simulink model "LateralControlDesignWashoutSystem"  (R2020b)
settings: Solver=ode15s  StartTime=0.0  StopTime=100  RelTol=1e-3
values from neighbouring files (symbols this model uses):
  actuatorDen = [1,   actuatorTimeConstant]    [LateralControl.m]    (also in LongitudinalControl.m)
  actuatorNum = actuatorGain*actuatorTimeConstant    (= 5)    [LateralControl.m]    (also in LongitudinalControl.m)
  DGain = PGain*Td    (= 0.156)    [LateralControl.m]    (also in LongitudinalControl.m = 0.0211)
  PGain = 1.56    [LateralControl.m]    (also in LongitudinalControl.m = 0.211)
  stepCommand = 0    [LateralControl.m]    (also in LongitudinalControl.m = 1)
undefined symbols (not defined in the file or in its folder): ALatWashOut, BLatWashOut, CLatWashOut, DLatWashOut, FRoll, FWashOut, InitialConditionsWashOut
libraries: slpidlib x2
settings Model: Creator=Antonis Kantounias  LastModifiedBy=Antonis Kantounias

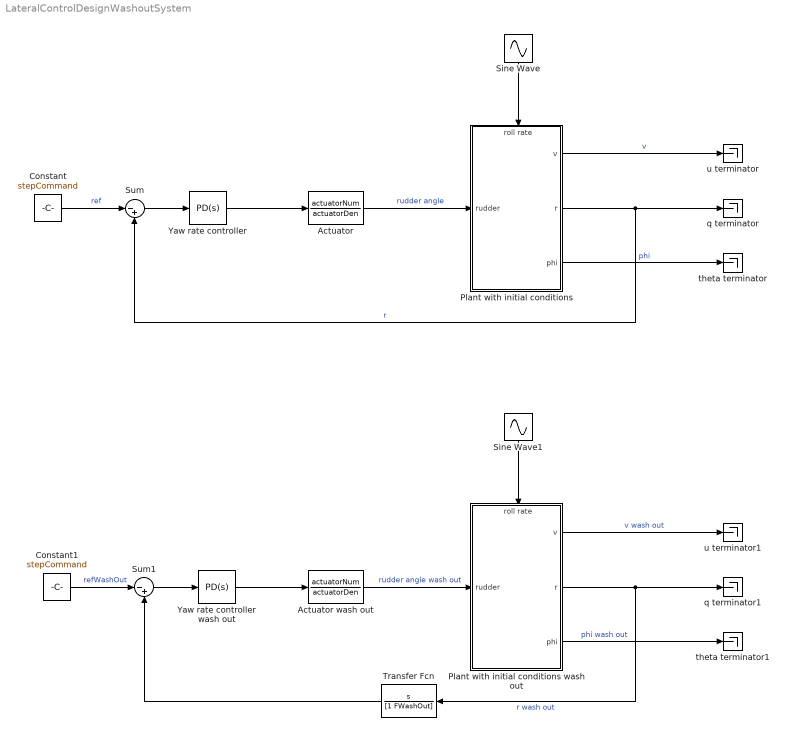
== system LateralControlDesignWashoutSystem ==
  Actuator : TransferFcn  Numerator=actuatorNum  Denominator=actuatorDen
  Actuator wash out : TransferFcn  Numerator=actuatorNum  Denominator=actuatorDen
  Constant : Constant  Value=stepCommand
  Constant1 : Constant  Value=stepCommand
  Plant with initial conditions : Subsystem
      settings: PortSchema="{\"entries\":[{\"content\":{\"sides\":[{\"content\":{\"connectorIds\":[\"In1\"]},\"type\":\"ConnectorPlacement.EquallySpacedRectSide\",\"uuid\":\"9289d697-068e-4568-8078-07f153e8e6b2\"},{\"content\":{\"connectorIds\":[\"Out1\",\"Out2\",\"Out3\"],\"side\":\"RIGHT\"},\"type\":\"ConnectorPlacement.EquallySpacedRectSide\",\"uuid\":\"07e3031a-d198-40ae-947d-4a1b1bfc261d\"},{\"content\":{\"connectorIds\":[\"In2\"],\"side\":\"TOP\"},\"type\":\"ConnectorPlacement.EquallySpacedRectSide\",\"uuid\":\"5510f47b-c9e9-4254-80f0-6c17108d1080\"},{\"content\":{\"connectorIds\":[],\"side\":\"HIDDEN\"},\"type\":\"ConnectorPlacement.EquallySpacedRectSide\",\"uuid\":\"028157a7-30e9-47c8-8173-f7276b1e18d8\"}]},\"type\":\"ConnectorPlacement.EquallySpacedConnector\",\"uuid\":\"3949036d-ff12-4955-8ea8-3a5b06263006\"}],\"packageUris\":[\"http://schema.mathworks.com/mf0/Connector/R2020b\"],\"version\":\"1.0\"}"
  Plant with initial conditions wash out : Subsystem
      settings: PortSchema="{\"entries\":[{\"content\":{\"sides\":[{\"content\":{\"connectorIds\":[\"In1\"]},\"type\":\"ConnectorPlacement.EquallySpacedRectSide\",\"uuid\":\"9289d697-068e-4568-8078-07f153e8e6b2\"},{\"content\":{\"connectorIds\":[\"Out1\",\"Out2\",\"Out3\"],\"side\":\"RIGHT\"},\"type\":\"ConnectorPlacement.EquallySpacedRectSide\",\"uuid\":\"07e3031a-d198-40ae-947d-4a1b1bfc261d\"},{\"content\":{\"connectorIds\":[\"In2\"],\"side\":\"TOP\"},\"type\":\"ConnectorPlacement.EquallySpacedRectSide\",\"uuid\":\"5510f47b-c9e9-4254-80f0-6c17108d1080\"},{\"content\":{\"connectorIds\":[],\"side\":\"HIDDEN\"},\"type\":\"ConnectorPlacement.EquallySpacedRectSide\",\"uuid\":\"028157a7-30e9-47c8-8173-f7276b1e18d8\"}]},\"type\":\"ConnectorPlacement.EquallySpacedConnector\",\"uuid\":\"3949036d-ff12-4955-8ea8-3a5b06263006\"}],\"packageUris\":[\"http://schema.mathworks.com/mf0/Connector/R2020b\"],\"version\":\"1.0\"}"
  Sine Wave : Sin  Frequency=FRoll  SampleTime=0
  Sine Wave1 : Sin  Frequency=FRoll  SampleTime=0
  Sum : Sum  Inputs=|-+
  Sum1 : Sum  Inputs=|-+
  Transfer Fcn : TransferFcn  Numerator=[1,0]  Denominator=[1 FWashOut]
  Yaw rate controller : slpidlib/PID Controller  Controller=PD  Form=Parallel  TimeDomain=Continuous-time  UseExternalTs=off  SampleTime=-1  IntegratorMethod=Forward Euler  FilterMethod=Forward Euler  ControllerParametersSource=internal  P=PGain  I=1  D=DGain  UseFilter=on  N=50  TunerSelectOption=Transfer Function Based (PID Tuner App)  InitialConditionSource=internal  InitialConditionForIntegrator=0  InitialConditionForFilter=0  DifferentiatorICPrevScaledInput=0  ExternalReset=none  TrackingMode=off  Kt=1  LimitOutput=off  SatLimitsSource=internal  UpperSaturationLimit=inf  LowerSaturationLimit=-inf  LinearizeAsGain=on  AntiWindupMode=none  Kb=1  POutMin=[]  POutMax=[]  IOutMin=[]  IOutMax=[]  DOutMin=[]  DOutMax=[]  NOutMin=[]  NOutMax=[]  SumOutMin=[]  SumOutMax=[]  SaturationOutMin=[]  SaturationOutMax=[]  PParamMin=[]  PParamMax=[]  IParamMin=[]  IParamMax=[]  DParamMin=[]  DParamMax=[]  NParamMin=[]  NParamMax=[]  KbParamMin=[]  KbParamMax=[]  KtParamMin=[]  KtParamMax=[]  KbOutMin=[]  KbOutMax=[]  KtOutMin=[]  KtOutMax=[]  IntegratorOutMin=[]  IntegratorOutMax=[]  FilterOutMin=[]  FilterOutMax=[]  SumI1OutMin=[]  SumI1OutMax=[]  SumI2OutMin=[]  SumI2OutMax=[]  SumI3OutMin=[]  SumI3OutMax=[]  SumI4OutMin=[]  SumI4OutMax=[]  SumDOutMin=[]  SumDOutMax=[]  DifferentiatorOutMin=[]  DifferentiatorOutMax=[]  FilterDiffOutCoefMin=[]  FilterDiffOutCoefMax=[]  ReciprocalOutMin=[]  ReciprocalOutMax=[]  SumDenOutMin=[]  SumDenOutMax=[]  SumNumOutMin=[]  SumNumOutMax=[]  DivideOutMin=[]  DivideOutMax=[]  UdiffTsProdOutMin=[]  UdiffTsProdOutMax=[]  NTsProdOutMin=[]  NTsProdOutMax=[]  UintegralTsProdOutMin=[]  UintegralTsProdOutMax=[]  UngainTsProdOutMin=[]  UngainTsProdOutMax=[]  IntegratorContinuousStateAttributes=''  IntegratorStateMustResolveToSignalObject=off  IntegratorRTWStateStorageClass=Auto  FilterContinuousStateAttributes=''  FilterStateMustResolveToSignalObject=off  FilterRTWStateStorageClass=Auto  ParallelPVariant=InternalParameters  IdealPVariant=Disabled  IVariant=Disabled  DVariant=InternalParameters  IntegratorVariant=Disabled  SatVariant=Disabled  AWVariant=Disabled  PCopyVariant=Disabled  TRVariant=Disabled  FdbkBlocksVariant=Forward  IdealPFdbkVariant=Disabled  SatFdbkVariant=Disabled  DerivativeFilterVariant=ContFilter  NVariant=InternalParameters  NCopyVariant=Disabled  FilterICVariant=InternalICsFilter  IntegratorICVariant=Disabled  ExternalResetVariant=Disabled  TRSumVariant=Passthrough  SumFdbkVariant=Disabled  SumVariant=Sum_PD  TsampFilterVariant=InternalTs  TsampNgainVariant=Passthrough  TsampIntegralVariant=Disabled_SignalSpec  ExternalSaturationOutDataTypeStr=Inherit: Same as second input
  "Yaw rate controller wash out " : slpidlib/PID Controller  Controller=PD  Form=Parallel  TimeDomain=Continuous-time  UseExternalTs=off  SampleTime=-1  IntegratorMethod=Forward Euler  FilterMethod=Forward Euler  ControllerParametersSource=internal  P=PGain  I=1  D=DGain  UseFilter=on  N=50  TunerSelectOption=Transfer Function Based (PID Tuner App)  InitialConditionSource=internal  InitialConditionForIntegrator=0  InitialConditionForFilter=0  DifferentiatorICPrevScaledInput=0  ExternalReset=none  TrackingMode=off  Kt=1  LimitOutput=off  SatLimitsSource=internal  UpperSaturationLimit=inf  LowerSaturationLimit=-inf  LinearizeAsGain=on  AntiWindupMode=none  Kb=1  POutMin=[]  POutMax=[]  IOutMin=[]  IOutMax=[]  DOutMin=[]  DOutMax=[]  NOutMin=[]  NOutMax=[]  SumOutMin=[]  SumOutMax=[]  SaturationOutMin=[]  SaturationOutMax=[]  PParamMin=[]  PParamMax=[]  IParamMin=[]  IParamMax=[]  DParamMin=[]  DParamMax=[]  NParamMin=[]  NParamMax=[]  KbParamMin=[]  KbParamMax=[]  KtParamMin=[]  KtParamMax=[]  KbOutMin=[]  KbOutMax=[]  KtOutMin=[]  KtOutMax=[]  IntegratorOutMin=[]  IntegratorOutMax=[]  FilterOutMin=[]  FilterOutMax=[]  SumI1OutMin=[]  SumI1OutMax=[]  SumI2OutMin=[]  SumI2OutMax=[]  SumI3OutMin=[]  SumI3OutMax=[]  SumI4OutMin=[]  SumI4OutMax=[]  SumDOutMin=[]  SumDOutMax=[]  DifferentiatorOutMin=[]  DifferentiatorOutMax=[]  FilterDiffOutCoefMin=[]  FilterDiffOutCoefMax=[]  ReciprocalOutMin=[]  ReciprocalOutMax=[]  SumDenOutMin=[]  SumDenOutMax=[]  SumNumOutMin=[]  SumNumOutMax=[]  DivideOutMin=[]  DivideOutMax=[]  UdiffTsProdOutMin=[]  UdiffTsProdOutMax=[]  NTsProdOutMin=[]  NTsProdOutMax=[]  UintegralTsProdOutMin=[]  UintegralTsProdOutMax=[]  UngainTsProdOutMin=[]  UngainTsProdOutMax=[]  IntegratorContinuousStateAttributes=''  IntegratorStateMustResolveToSignalObject=off  IntegratorRTWStateStorageClass=Auto  FilterContinuousStateAttributes=''  FilterStateMustResolveToSignalObject=off  FilterRTWStateStorageClass=Auto  ParallelPVariant=InternalParameters  IdealPVariant=Disabled  IVariant=Disabled  DVariant=InternalParameters  IntegratorVariant=Disabled  SatVariant=Disabled  AWVariant=Disabled  PCopyVariant=Disabled  TRVariant=Disabled  FdbkBlocksVariant=Forward  IdealPFdbkVariant=Disabled  SatFdbkVariant=Disabled  DerivativeFilterVariant=ContFilter  NVariant=InternalParameters  NCopyVariant=Disabled  FilterICVariant=InternalICsFilter  IntegratorICVariant=Disabled  ExternalResetVariant=Disabled  TRSumVariant=Passthrough  SumFdbkVariant=Disabled  SumVariant=Sum_PD  TsampFilterVariant=InternalTs  TsampNgainVariant=Passthrough  TsampIntegralVariant=Disabled_SignalSpec  ExternalSaturationOutDataTypeStr=Inherit: Same as second input
  q terminator : Terminator
  q terminator1 : Terminator
  theta terminator : Terminator
  theta terminator1 : Terminator
  u terminator : Terminator
  u terminator1 : Terminator
  wires:
  Plant with initial conditions/2(r) -> q terminator/1, Sum/2  "r"
  Plant with initial conditions/1(v) -> u terminator/1  "v"
  Plant with initial conditions/3(phi) -> theta terminator/1  "phi"
  Constant/1 -> Sum/1  "ref"
  Sum/1 -> Yaw rate controller/1
  Yaw rate controller/1 -> Actuator/1
  Actuator/1 -> Plant with initial conditions/1(rudder)  "rudder angle"
  Sine Wave/1 -> Plant with initial conditions/2(roll rate)
  Sine Wave1/1 -> Plant with initial conditions wash out/2(roll rate)
  Actuator wash out/1 -> Plant with initial conditions wash out/1(rudder)  "rudder angle wash out"
  "Yaw rate controller wash out "/1 -> Actuator wash out/1
  Sum1/1 -> "Yaw rate controller wash out "/1
  Constant1/1 -> Sum1/1  "refWashOut"
  Plant with initial conditions wash out/3(phi) -> theta terminator1/1  "phi wash out"
  Plant with initial conditions wash out/1(v) -> u terminator1/1  "v wash out"
  Plant with initial conditions wash out/2(r) -> Transfer Fcn/1, q terminator1/1  "r wash out"
  Transfer Fcn/1 -> Sum1/2

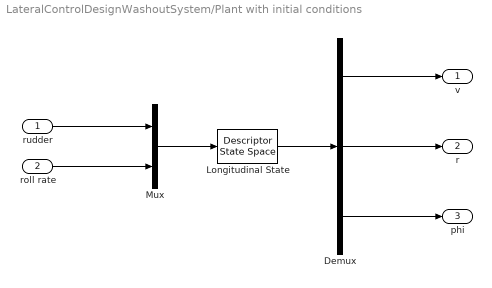
== system LateralControlDesignWashoutSystem/Plant with initial conditions ==
  rudder : Inport
  roll rate : Inport  Port=2
  Demux : Demux  Outputs=3
  "Longitudinal State " : DescriptorStateSpace  E=ELatWashOut  A=ALatWashOut  B=BLatWashOut  C=CLatWashOut  D=DLatWashOut  InitialCondition=InitialConditionsWashOut  ContinuousStateAttributes='LateralSystem'
  Mux : Mux  Inputs=2
  v : Outport
  r : Outport  Port=2
  phi : Outport  Port=3
  wires:
  "Longitudinal State "/1 -> Demux/1
  Demux/3 -> phi/1
  rudder/1 -> Mux/1
  roll rate/1 -> Mux/2
  Mux/1 -> "Longitudinal State "/1
  Demux/2 -> r/1
  Demux/1 -> v/1

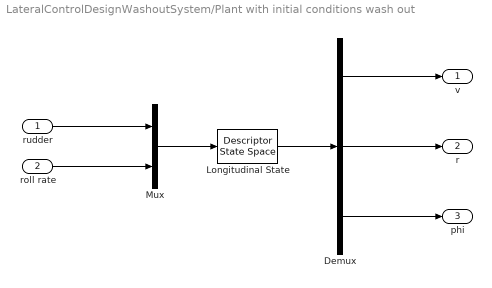
== system LateralControlDesignWashoutSystem/Plant with initial conditions wash out ==
  rudder : Inport
  roll rate : Inport  Port=2
  Demux : Demux  Outputs=3
  "Longitudinal State " : DescriptorStateSpace  E=ELatWashOut  A=ALatWashOut  B=BLatWashOut  C=CLatWashOut  D=DLatWashOut  InitialCondition=InitialConditionsWashOut  ContinuousStateAttributes='LateralSystem'
  Mux : Mux  Inputs=2
  v : Outport
  r : Outport  Port=2
  phi : Outport  Port=3
  wires:
  Demux/1 -> v/1
  Demux/2 -> r/1
  Mux/1 -> "Longitudinal State "/1
  roll rate/1 -> Mux/2
  rudder/1 -> Mux/1
  Demux/3 -> phi/1
  "Longitudinal State "/1 -> Demux/1
